simulink model "sim_tcst_2024_att_ctrl"  (R2020a)
settings: Solver=ode4  StartTime=0.0  StopTime=30.0  FixedStep=0.01  RelTol=1e-3
values from neighbouring files (symbols this model uses):
  beta0 = 2    [init_tcst_2024_att_ctrl.m]
  c1_diff_sigma_bar_w = diag([12; 12; 12])    [init_tcst_2024_att_ctrl.m]
  c1_diff_ui = diag([25; 30; 20])    [init_tcst_2024_att_ctrl.m]
  c2_diff_sigma_bar_w = diag([12; 12; 12])    [init_tcst_2024_att_ctrl.m]
  c2_diff_ui = diag([50; 50; 10])    [init_tcst_2024_att_ctrl.m]
  c3_diff_sigma_bar_w = diag([15; 15; 15])    [init_tcst_2024_att_ctrl.m]
  c3_diff_ui = diag([15; 15; 10])    [init_tcst_2024_att_ctrl.m]
  dw_aa_t = 0.2 * ones(3, 5) + ( 1.0 - 0.2 ) * rand(3, 5)    [init_tcst_2024_att_ctrl.m]
  dw_ff_t = [ 0.4 * ones(1, 5) + ( 1.0 - 0.4 ) * rand(1, 5);                      0.4 * ones(1, 5) + ( 1.0 - 0.4 ) * rand(1, 5);                      0.2 * ones(1, 5) + ( 0.6 - 0.2 ) * rand(1, 5) ]    [init_tcst_2024_att_ctrl.m]
  dw_phi_t = ( - pi / 2 ) * ones(3, 5) + ( pi / 2 - ( - pi / 2 ) ) * rand(3, 5)    [init_tcst_2024_att_ctrl.m]
  dwci_init = zeros(3,5)    [init_tcst_2024_att_ctrl.m]
  err_Ri_bar_init = zeros(3,NF)    [init_tcst_2024_att_ctrl.m]
  Fi_init = zeros(3,NF)    [init_tcst_2024_att_ctrl.m]
  h1w = diag([20.0; 20.0; 20.0])    [init_tcst_2024_att_ctrl.m]
  h2w = diag([30.0; 35.0; 35.0])    [init_tcst_2024_att_ctrl.m]
  h3w = diag([30.0; 25.0; 30.0])    [init_tcst_2024_att_ctrl.m]
  Ji = zeros(3,3,NF)    [init_tcst_2024_att_ctrl.m]
  kr1 = 10    [init_tcst_2024_att_ctrl.m]
  kr2 = 10    [init_tcst_2024_att_ctrl.m]
  kr3 = 5    [init_tcst_2024_att_ctrl.m]
  Lamd_diff_sigma_bar_w = 0.8    [init_tcst_2024_att_ctrl.m]
  Lamd_diff_ui = 0.8    [init_tcst_2024_att_ctrl.m]
  mu_d_w = 100    [init_tcst_2024_att_ctrl.m]
  pos0 = zeros(3, 1)    [init_tcst_2024_att_ctrl.m]
  PZ0 = P0(3)    [init_tcst_2024_att_ctrl.m]
  PZ1 = 10    [init_tcst_2024_att_ctrl.m]
  Qci_init = repmat([1;0;0;0],1,NF)    [init_tcst_2024_att_ctrl.m]
  Qei_init = zeros(4,NF)    [init_tcst_2024_att_ctrl.m]
  R0 = 4    [init_tcst_2024_att_ctrl.m]
  R1 = 8    [init_tcst_2024_att_ctrl.m]
  Rci_init = zeros(3,3,NF)    [init_tcst_2024_att_ctrl.m]
  Rei_init = zeros(3,3,NF)    [init_tcst_2024_att_ctrl.m]
  Ri_init = zeros(3,3,NF)    [init_tcst_2024_att_ctrl.m]
  Rx2 = 10    [init_tcst_2024_att_ctrl.m]
  Ry2 = 6    [init_tcst_2024_att_ctrl.m]
  Rz2 = 4    [init_tcst_2024_att_ctrl.m]
  T0 = 0    [init_tcst_2024_att_ctrl.m]
  T1 = tseq1    (= 10)    [init_tcst_2024_att_ctrl.m]
  T2 = tseq1 + tseq12 + tseq2    (= 30)    [init_tcst_2024_att_ctrl.m]
  ui_init = zeros(3,NF)    [init_tcst_2024_att_ctrl.m]
  V_Phi_Rei_init = zeros(3,NF)    [init_tcst_2024_att_ctrl.m]
  vel0 = zeros(3, 1)    [init_tcst_2024_att_ctrl.m]
  wci_init = zeros(3,5)    [init_tcst_2024_att_ctrl.m]
  wei_init = zeros(3,NF)    [init_tcst_2024_att_ctrl.m]
  zeta_diff_sigma_bar_w = 0.3    [init_tcst_2024_att_ctrl.m]
  zeta_diff_ui = 0.05    [init_tcst_2024_att_ctrl.m]
undefined symbols (not defined in the file or in its folder): cal_frac_squ, p_alfaw1, p_alfaw2, q_alfaw1, q_alfaw2, Qi_init, wi_init
(part 3 of 4)

== matlab function sim_tcst_2024_att_ctrl/combine wci dwci ==
  data: wci_node_1 input; wci_vec output; wci_node_2 input; wci_node_3 input; wci_node_4 input; wci_node_5 input; dwci_vec output; dwci_node_1 input; dwci_node_2 input; dwci_node_3 input; dwci_node_4 input; dwci_node_5 input
function [wci_vec, dwci_vec] = fcn(wci_node_1, wci_node_2, wci_node_3, wci_node_4, wci_node_5, ...
                                                                dwci_node_1, dwci_node_2, dwci_node_3, dwci_node_4, dwci_node_5)
%%%% 合并姿态角速率指令及其导数
wci_vec = [wci_node_1(:), wci_node_2(:), wci_node_3(:), wci_node_4(:), wci_node_5(:)];
dwci_vec = [dwci_node_1(:), dwci_node_2(:), dwci_node_3(:), dwci_node_4(:), dwci_node_5(:)];

== matlab function sim_tcst_2024_att_ctrl/cal abs 11 ==
  data: x input; y output
function y = fcn(x)
y = abs(x(:));

== matlab function sim_tcst_2024_att_ctrl/cal abs 12 ==
  data: x input; y output
function y = fcn(x)
y = abs(x(:));

== matlab function sim_tcst_2024_att_ctrl/cal abs 13 ==
  data: x input; y output
function y = fcn(x)
y = abs(x(:));

== matlab function sim_tcst_2024_att_ctrl/cal abs 14 ==
  data: x input; y output
function y = fcn(x)
y = abs(x(:));

== matlab function sim_tcst_2024_att_ctrl/cal abs 15 ==
  data: x input; y output
function y = fcn(x)
y = abs(x(:));

== matlab function sim_tcst_2024_att_ctrl/cal err_Ri_bar agent 1 ==
  data: kr1 input; err_Ri_bar_1 output; wei_vec input; V_Phi_Rei_vec input
function err_Ri_bar_1 = fcn(kr1, wei_vec, V_Phi_Rei_vec)
%%%% 计算辅助姿态旋转误差
iiuav = 1;
err_Ri_bar_1 = wei_vec(:,iiuav) + kr1 * V_Phi_Rei_vec(:,iiuav);
end

== matlab function sim_tcst_2024_att_ctrl/cal abs 16 ==
  data: x input; y output
function y = fcn(x)
y = abs(x(:));

== matlab function sim_tcst_2024_att_ctrl/cal abs 17 ==
  data: x input; y output
function y = fcn(x)
y = abs(x(:));

== matlab function sim_tcst_2024_att_ctrl/cal abs 18 ==
  data: x input; y output
function y = fcn(x)
y = abs(x(:));

== matlab function sim_tcst_2024_att_ctrl/combine tau ==
  data: tau_1 input; taui_vec output; tau_2 input; tau_3 input; tau_4 input; tau_5 input
function taui_vec = fcn(tau_1, tau_2, tau_3, tau_4, tau_5)
%%%% 合并辅助姿态角速率
taui_vec = [tau_1(:), tau_2(:), tau_3(:), tau_4(:), tau_5(:)];

== matlab function sim_tcst_2024_att_ctrl/wi dynam agent 1 ==
  data: Ji input; dwi_1 output; wi_vec input; taui_vec input; dw_vec input
function dwi_1 = fcn(Ji, wi_vec, taui_vec, dw_vec)
%%%% 更新姿态角速率微分方程
iiuav = 1;
dwi_1 = inv(Ji(:,:,iiuav)) * ( -cal_askew_mat(wi_vec(:,iiuav)) * Ji(:,:,iiuav) * wi_vec(:,iiuav) ... 
                                                + taui_vec(:,iiuav) + dw_vec(:,iiuav) );

end

== matlab function sim_tcst_2024_att_ctrl/cal abs 19 ==
  data: x input; y output
function y = fcn(x)
y = abs(x(:));

== matlab function sim_tcst_2024_att_ctrl/cal abs 20 ==
  data: x input; y output
function y = fcn(x)
y = abs(x(:));

== matlab function sim_tcst_2024_att_ctrl/cal d_sigma_w agent 1 ==
  data: h3w input; d_sigma_w_1 output; Ji input; wi_vec input; taui_vec input; sigma_w_bar_vec input
function d_sigma_w_1 = fcn(h3w, Ji, wi_vec, taui_vec, sigma_w_bar_vec)
%%%% 计算辅助姿态角速率导数
iiuav = 1;
d_sigma_w_1 = inv(Ji(:,:,iiuav)) * ( -cal_askew_mat(wi_vec(:,iiuav)) * Ji(:,:,iiuav) * wi_vec(:,iiuav) ...
                            + taui_vec(:,iiuav) + h3w * sigma_w_bar_vec(:,iiuav) );

== matlab function sim_tcst_2024_att_ctrl/cal d_sigma_w agent 2 ==
  data: h3w input; d_sigma_w_2 output; Ji input; wi_vec input; taui_vec input; sigma_w_bar_vec input
function d_sigma_w_2 = fcn(h3w, Ji, wi_vec, taui_vec, sigma_w_bar_vec)
%%%% 计算辅助姿态角速率导数
iiuav = 2;
d_sigma_w_2 = inv(Ji(:,:,iiuav)) * ( -cal_askew_mat(wi_vec(:,iiuav)) * Ji(:,:,iiuav) * wi_vec(:,iiuav) ...
                            + taui_vec(:,iiuav) + h3w * sigma_w_bar_vec(:,iiuav) );

== matlab function sim_tcst_2024_att_ctrl/cal d_sigma_w agent 3 ==
  data: h3w input; d_sigma_w_3 output; Ji input; wi_vec input; taui_vec input; sigma_w_bar_vec input
function d_sigma_w_3 = fcn(h3w, Ji, wi_vec, taui_vec, sigma_w_bar_vec)
%%%% 计算辅助姿态角速率导数
iiuav = 3;
d_sigma_w_3 = inv(Ji(:,:,iiuav)) * ( -cal_askew_mat(wi_vec(:,iiuav)) * Ji(:,:,iiuav) * wi_vec(:,iiuav) ...
                            + taui_vec(:,iiuav) + h3w * sigma_w_bar_vec(:,iiuav) );

== matlab function sim_tcst_2024_att_ctrl/cal err_Ri_bar agent 2 ==
  data: kr1 input; err_Ri_bar_2 output; wei_vec input; V_Phi_Rei_vec input
function err_Ri_bar_2 = fcn(kr1, wei_vec, V_Phi_Rei_vec)
%%%% 计算辅助姿态旋转误差
iiuav = 2;
err_Ri_bar_2 = wei_vec(:,iiuav) + kr1 * V_Phi_Rei_vec(:,iiuav);
end

== matlab function sim_tcst_2024_att_ctrl/cal d_sigma_w agent 4 ==
  data: h3w input; d_sigma_w_4 output; Ji input; wi_vec input; taui_vec input; sigma_w_bar_vec input
function d_sigma_w_4 = fcn(h3w, Ji, wi_vec, taui_vec, sigma_w_bar_vec)
%%%% 计算辅助姿态角速率导数
iiuav = 4;
d_sigma_w_4 = inv(Ji(:,:,iiuav)) * ( -cal_askew_mat(wi_vec(:,iiuav)) * Ji(:,:,iiuav) * wi_vec(:,iiuav) ...
                            + taui_vec(:,iiuav) + h3w * sigma_w_bar_vec(:,iiuav) );

== matlab function sim_tcst_2024_att_ctrl/wi dynam agent 2 ==
  data: Ji input; dwi_2 output; wi_vec input; taui_vec input; dw_vec input
function dwi_2 = fcn(Ji, wi_vec, taui_vec, dw_vec)
%%%% 更新姿态角速率微分方程
iiuav = 2;
dwi_2 = inv(Ji(:,:,iiuav)) * ( -cal_askew_mat(wi_vec(:,iiuav)) * Ji(:,:,iiuav) * wi_vec(:,iiuav) ... 
                                                + taui_vec(:,iiuav) + dw_vec(:,iiuav) );

end

== matlab function sim_tcst_2024_att_ctrl/wi dynam agent 3 ==
  data: Ji input; dwi_3 output; wi_vec input; taui_vec input; dw_vec input
function dwi_3 = fcn(Ji, wi_vec, taui_vec, dw_vec)
%%%% 更新姿态角速率微分方程
iiuav = 3;
dwi_3 = inv(Ji(:,:,iiuav)) * ( -cal_askew_mat(wi_vec(:,iiuav)) * Ji(:,:,iiuav) * wi_vec(:,iiuav) ...
                                                + taui_vec(:,iiuav) + dw_vec(:,iiuav) );

end

== matlab function sim_tcst_2024_att_ctrl/wi dynam agent 4 ==
  data: Ji input; dwi_4 output; wi_vec input; taui_vec input; dw_vec input
function dwi_4 = fcn(Ji, wi_vec, taui_vec, dw_vec)
%%%% 更新姿态角速率微分方程
iiuav = 4;
dwi_4 = inv(Ji(:,:,iiuav)) * ( -cal_askew_mat(wi_vec(:,iiuav)) * Ji(:,:,iiuav) * wi_vec(:,iiuav) ...
                                                + taui_vec(:,iiuav) + dw_vec(:,iiuav) );

end

== matlab function sim_tcst_2024_att_ctrl/wi dynam agent 5 ==
  data: Ji input; dwi_5 output; wi_vec input; taui_vec input; dw_vec input
function dwi_5 = fcn(Ji, wi_vec, taui_vec, dw_vec)
%%%% 更新姿态角速率微分方程
iiuav = 5;
dwi_5 = inv(Ji(:,:,iiuav)) * ( -cal_askew_mat(wi_vec(:,iiuav)) * Ji(:,:,iiuav) * wi_vec(:,iiuav) ...
                                                + taui_vec(:,iiuav) + dw_vec(:,iiuav) );

end

== matlab function sim_tcst_2024_att_ctrl/combine dwi ==
  data: wi_1 input; wi_vec output; wi_2 input; wi_3 input; wi_4 input; wi_5 input
function wi_vec = fcn(wi_1, wi_2, wi_3, wi_4, wi_5)
%%%% 合并姿态角速率
wi_vec = [wi_1(:), wi_2(:), wi_3(:), wi_4(:), wi_5(:)];

== matlab function sim_tcst_2024_att_ctrl/Qi dynam agent 1 ==
  data: Qi_vec input; dQi_1 output; wi_vec input
function dQi_1 = fcn(Qi_vec, wi_vec)
%%%% 更新四元数微分方程
iiuav = 1;

wi = wi_vec(:,iiuav);
thetai = Qi_vec(1,iiuav);
qi = Qi_vec(2:4,iiuav);

GammaQi = zeros(4,3);
GammaQi(1,:) = -(qi');
GammaQi(2:4,:) = thetai*eye(3,3) + cal_askew_mat(qi);
dQi_1 = (1/2)*GammaQi*wi;

end

== matlab function sim_tcst_2024_att_ctrl/Qi dynam agent 2 ==
  data: Qi_vec input; dQi_2 output; wi_vec input
function dQi_2 = fcn(Qi_vec, wi_vec)
%%%% 更新四元数微分方程
iiuav = 2;

wi = wi_vec(:,iiuav);
thetai = Qi_vec(1,iiuav);
qi = Qi_vec(2:4,iiuav);

GammaQi = zeros(4,3);
GammaQi(1,:) = -(qi');
GammaQi(2:4,:) = thetai*eye(3,3) + cal_askew_mat(qi);
dQi_2 = (1/2)*GammaQi*wi;

end

== matlab function sim_tcst_2024_att_ctrl/cal d_sigma_w agent 5 ==
  data: h3w input; d_sigma_w_5 output; Ji input; wi_vec input; taui_vec input; sigma_w_bar_vec input
function d_sigma_w_5 = fcn(h3w, Ji, wi_vec, taui_vec, sigma_w_bar_vec)
%%%% 计算辅助姿态角速率导数
iiuav = 5;
d_sigma_w_5 = inv(Ji(:,:,iiuav)) * ( -cal_askew_mat(wi_vec(:,iiuav)) * Ji(:,:,iiuav) * wi_vec(:,iiuav) ...
                            + taui_vec(:,iiuav) + h3w * sigma_w_bar_vec(:,iiuav) );

== matlab function sim_tcst_2024_att_ctrl/cal err_Ri_bar agent 3 ==
  data: kr1 input; err_Ri_bar_3 output; wei_vec input; V_Phi_Rei_vec input
function err_Ri_bar_3 = fcn(kr1, wei_vec, V_Phi_Rei_vec)
%%%% 计算辅助姿态旋转误差
iiuav = 3;
err_Ri_bar_3 = wei_vec(:,iiuav) + kr1 * V_Phi_Rei_vec(:,iiuav);
end

== matlab function sim_tcst_2024_att_ctrl/cal differentiator d_sigma_bar_w_hat agent 1/cal differentiator ==
  data: c1 input; d_sigma_bar_v_hat output; d_dsigma_bar_v_hat output; d_d2sigma_bar_v_hat output; c2 input; c3 input; chi_t input; sigma_bar_v_sig_1 input; sigma_bar_v_sig_2 input; sigma_bar_v_sig_3 input; sigma_bar_v_sig_4 input; sigma_bar_v_sig_5 input; sigma_bar_v_sig_6 input; d_sigma_bar_v_hat input; d2_sigma_bar_v_hat input
function [d_sigma_bar_v_hat, d_dsigma_bar_v_hat, d_d2sigma_bar_v_hat] = fcn(c1, c2, c3, chi_t, sigma_bar_v_sig_1, sigma_bar_v_sig_2, sigma_bar_v_sig_3, ...
                                                                                                                                                sigma_bar_v_sig_4, sigma_bar_v_sig_5, sigma_bar_v_sig_6, d_sigma_bar_v_hat, d2_sigma_bar_v_hat)
d_d2sigma_bar_v_hat = -chi_t .* c1 * sigma_bar_v_sig_1(:) - (1 - chi_t) .* c1 * sigma_bar_v_sig_2(:);
d_dsigma_bar_v_hat = -chi_t .* c2 * sigma_bar_v_sig_3(:) - (1 - chi_t) .* c2 * sigma_bar_v_sig_4(:) + d2_sigma_bar_v_hat(:);
d_sigma_bar_v_hat = -chi_t .* c3 * sigma_bar_v_sig_5(:) - (1 - chi_t) .* c3 * sigma_bar_v_sig_6(:) + d_sigma_bar_v_hat(:);

== matlab function sim_tcst_2024_att_ctrl/cal differentiator d_sigma_bar_w_hat agent 1/cal sig ==
  data: x input; z output; y input
function z = fcn(x, y)
z = x(:) .* sign(y(:));

== matlab function sim_tcst_2024_att_ctrl/cal differentiator d_sigma_bar_w_hat agent 1/cal sig1 ==
  data: x input; z output; y input
function z = fcn(x, y)
z = x(:) .* sign(y(:));

== matlab function sim_tcst_2024_att_ctrl/cal differentiator d_sigma_bar_w_hat agent 1/cal sig2 ==
  data: x input; z output; y input
function z = fcn(x, y)
z = x(:) .* sign(y(:));

== matlab function sim_tcst_2024_att_ctrl/cal differentiator d_sigma_bar_w_hat agent 1/cal sig3 ==
  data: x input; z output; y input
function z = fcn(x, y)
z = x(:) .* sign(y(:));

== matlab function sim_tcst_2024_att_ctrl/cal differentiator d_sigma_bar_w_hat agent 1/cal sig4 ==
  data: x input; z output; y input
function z = fcn(x, y)
z = x(:) .* sign(y(:));

== matlab function sim_tcst_2024_att_ctrl/cal differentiator d_sigma_bar_w_hat agent 1/cal sig5 ==
  data: x input; z output; y input
function z = fcn(x, y)
z = x(:) .* sign(y(:));

== matlab function sim_tcst_2024_att_ctrl/cal differentiator d_sigma_bar_w_hat agent 1/choose sigma_bar_w ==
  data: x input; y output
function y = fcn(x)
iiuav = 1;
y = x(:,iiuav);

== matlab function sim_tcst_2024_att_ctrl/cal differentiator d_sigma_bar_w_hat agent 1/trans to column20 ==
  data: x input; y output
function y = fcn(x)
y = x(:);

== matlab function sim_tcst_2024_att_ctrl/cal differentiator d_sigma_bar_w_hat agent 1/trans to column21 ==
  data: x input; y output
function y = fcn(x)
y = x(:);

== matlab function sim_tcst_2024_att_ctrl/cal err_Ri_bar agent 4 ==
  data: kr1 input; err_Ri_bar_4 output; wei_vec input; V_Phi_Rei_vec input
function err_Ri_bar_4 = fcn(kr1, wei_vec, V_Phi_Rei_vec)
%%%% 计算辅助姿态旋转误差
iiuav = 4;
err_Ri_bar_4 = wei_vec(:,iiuav) + kr1 * V_Phi_Rei_vec(:,iiuav);
end

== matlab function sim_tcst_2024_att_ctrl/cal differentiator d_sigma_bar_w_hat agent 1/trans to column22 ==
  data: x input; y output
function y = fcn(x)
y = x(:);

== matlab function sim_tcst_2024_att_ctrl/cal differentiator d_sigma_bar_w_hat agent 1/trans to column23 ==
  data: x input; y output
function y = fcn(x)
y = x(:);

== matlab function sim_tcst_2024_att_ctrl/cal differentiator d_sigma_bar_w_hat agent 1/trans to column24 ==
  data: x input; y output
function y = fcn(x)
y = x(:);

== matlab function sim_tcst_2024_att_ctrl/cal differentiator d_sigma_bar_w_hat agent 1/trans to column25 ==
  data: x input; y output
function y = fcn(x)
y = x(:);

== matlab function sim_tcst_2024_att_ctrl/cal differentiator d_sigma_bar_w_hat agent 2/cal differentiator ==
  data: c1 input; d_sigma_bar_v_hat output; d_dsigma_bar_v_hat output; d_d2sigma_bar_v_hat output; c2 input; c3 input; chi_t input; sigma_bar_v_sig_1 input; sigma_bar_v_sig_2 input; sigma_bar_v_sig_3 input; sigma_bar_v_sig_4 input; sigma_bar_v_sig_5 input; sigma_bar_v_sig_6 input; d_sigma_bar_v_hat input; d2_sigma_bar_v_hat input
function [d_sigma_bar_v_hat, d_dsigma_bar_v_hat, d_d2sigma_bar_v_hat] = fcn(c1, c2, c3, chi_t, sigma_bar_v_sig_1, sigma_bar_v_sig_2, sigma_bar_v_sig_3, ...
                                                                                                                                                sigma_bar_v_sig_4, sigma_bar_v_sig_5, sigma_bar_v_sig_6, d_sigma_bar_v_hat, d2_sigma_bar_v_hat)
d_d2sigma_bar_v_hat = -chi_t .* c1 * sigma_bar_v_sig_1(:) - (1 - chi_t) .* c1 * sigma_bar_v_sig_2(:);
d_dsigma_bar_v_hat = -chi_t .* c2 * sigma_bar_v_sig_3(:) - (1 - chi_t) .* c2 * sigma_bar_v_sig_4(:) + d2_sigma_bar_v_hat(:);
d_sigma_bar_v_hat = -chi_t .* c3 * sigma_bar_v_sig_5(:) - (1 - chi_t) .* c3 * sigma_bar_v_sig_6(:) + d_sigma_bar_v_hat(:);

== matlab function sim_tcst_2024_att_ctrl/cal differentiator d_sigma_bar_w_hat agent 2/cal sig ==
  data: x input; z output; y input
function z = fcn(x, y)
z = x(:) .* sign(y(:));

== matlab function sim_tcst_2024_att_ctrl/cal differentiator d_sigma_bar_w_hat agent 2/cal sig1 ==
  data: x input; z output; y input
function z = fcn(x, y)
z = x(:) .* sign(y(:));

== matlab function sim_tcst_2024_att_ctrl/cal differentiator d_sigma_bar_w_hat agent 2/cal sig2 ==
  data: x input; z output; y input
function z = fcn(x, y)
z = x(:) .* sign(y(:));

== matlab function sim_tcst_2024_att_ctrl/cal differentiator d_sigma_bar_w_hat agent 2/cal sig3 ==
  data: x input; z output; y input
function z = fcn(x, y)
z = x(:) .* sign(y(:));

== matlab function sim_tcst_2024_att_ctrl/cal differentiator d_sigma_bar_w_hat agent 2/cal sig4 ==
  data: x input; z output; y input
function z = fcn(x, y)
z = x(:) .* sign(y(:));

== matlab function sim_tcst_2024_att_ctrl/cal differentiator d_sigma_bar_w_hat agent 2/cal sig5 ==
  data: x input; z output; y input
function z = fcn(x, y)
z = x(:) .* sign(y(:));

== matlab function sim_tcst_2024_att_ctrl/depart wc5 ==
  data: y output; x input
function y = fcn(x)
y = x(:,5);

end

== matlab function sim_tcst_2024_att_ctrl/cal differentiator d_sigma_bar_w_hat agent 2/choose sigma_bar_w ==
  data: x input; y output
function y = fcn(x)
iiuav = 2;
y = x(:,iiuav);

== matlab function sim_tcst_2024_att_ctrl/cal differentiator d_sigma_bar_w_hat agent 2/trans to column20 ==
  data: x input; y output
function y = fcn(x)
y = x(:);

== matlab function sim_tcst_2024_att_ctrl/cal differentiator d_sigma_bar_w_hat agent 2/trans to column21 ==
  data: x input; y output
function y = fcn(x)
y = x(:);

== matlab function sim_tcst_2024_att_ctrl/cal differentiator d_sigma_bar_w_hat agent 2/trans to column22 ==
  data: x input; y output
function y = fcn(x)
y = x(:);

== matlab function sim_tcst_2024_att_ctrl/cal differentiator d_sigma_bar_w_hat agent 2/trans to column23 ==
  data: x input; y output
function y = fcn(x)
y = x(:);

== matlab function sim_tcst_2024_att_ctrl/cal taui agent 1 ==
  data: kr1 input; kr2 input; kr3 input; tau_1 output; Ji input; wi_vec input; wei_vec input; err_Ri_bar_vec input; Fi_vec input; VTi_vec input; dw_hat_vec input
function tau_1 = fcn(kr1, kr2, kr3, Ji, wi_vec, wei_vec, err_Ri_bar_vec, Fi_vec, VTi_vec, dw_hat_vec)
%%%% 计算用于姿态控制的驱动力矩控制输入
iiuav = 1;
tau_1 = -( kr3 + kr2 ) * err_Ri_bar_vec(:,iiuav) - kr1 * Ji(:,:,iiuav) * wei_vec(:,iiuav) ...
                + cal_askew_mat( wi_vec(:,iiuav) ) * Ji(:,:,iiuav) * wi_vec(:,iiuav) ...
                - Ji(:,:,iiuav) * Fi_vec(:,iiuav) - dw_hat_vec(:,iiuav) - VTi_vec(:,iiuav);
end

== matlab function sim_tcst_2024_att_ctrl/Qi dynam agent 3 ==
  data: Qi_vec input; dQi_3 output; wi_vec input
function dQi_3 = fcn(Qi_vec, wi_vec)
%%%% 更新四元数微分方程
iiuav = 3;

wi = wi_vec(:,iiuav);
thetai = Qi_vec(1,iiuav);
qi = Qi_vec(2:4,iiuav);

GammaQi = zeros(4,3);
GammaQi(1,:) = -(qi');
GammaQi(2:4,:) = thetai*eye(3,3) + cal_askew_mat(qi);
dQi_3 = (1/2)*GammaQi*wi;

end

== matlab function sim_tcst_2024_att_ctrl/Qi dynam agent 4 ==
  data: Qi_vec input; dQi_4 output; wi_vec input
function dQi_4 = fcn(Qi_vec, wi_vec)
%%%% 更新四元数微分方程
iiuav = 4;

wi = wi_vec(:,iiuav);
thetai = Qi_vec(1,iiuav);
qi = Qi_vec(2:4,iiuav);

GammaQi = zeros(4,3);
GammaQi(1,:) = -(qi');
GammaQi(2:4,:) = thetai*eye(3,3) + cal_askew_mat(qi);
dQi_4 = (1/2)*GammaQi*wi;

end

== matlab function sim_tcst_2024_att_ctrl/depart wc1 ==
  data: y output; x input
function y = fcn(x)
y = x(:,1);

end

== matlab function sim_tcst_2024_att_ctrl/Qi dynam agent 5 ==
  data: Qi_vec input; dQi_5 output; wi_vec input
function dQi_5 = fcn(Qi_vec, wi_vec)
%%%% 更新四元数微分方程
iiuav = 5;

wi = wi_vec(:,iiuav);
thetai = Qi_vec(1,iiuav);
qi = Qi_vec(2:4,iiuav);

GammaQi = zeros(4,3);
GammaQi(1,:) = -(qi');
GammaQi(2:4,:) = thetai*eye(3,3) + cal_askew_mat(qi);
dQi_5 = (1/2)*GammaQi*wi;

end

== matlab function sim_tcst_2024_att_ctrl/combine Qi Ri ==
  data: Qi_1 input; Qi_vec output; Qi_2 input; Qi_3 input; Qi_4 input; Qi_5 input; Ri_1 input; Ri_2 input; Ri_3 input; Ri_4 input; Ri_5 input; Ri_vec output
function [Qi_vec, Ri_vec] = fcn(Qi_1, Qi_2, Qi_3, Qi_4, Qi_5, ...
                                                        Ri_1, Ri_2, Ri_3, Ri_4, Ri_5)
%%%% 合并四元数和姿态旋转矩阵
Qi_vec = zeros(4,5);
Qi_vec(:,1) = Qi_1(:);
Qi_vec(:,2) = Qi_2(:);
Qi_vec(:,3) = Qi_3(:);
Qi_vec(:,4) = Qi_4(:);
Qi_vec(:,5) = Qi_5(:);

Ri_vec = zeros(3,3,5);
Ri_vec(:,:,1) = Ri_1;
Ri_vec(:,:,2) = Ri_2;
Ri_vec(:,:,3) = Ri_3;
Ri_vec(:,:,4) = Ri_4;
Ri_vec(:,:,5) = Ri_5;

== matlab function sim_tcst_2024_att_ctrl/cal differentiator d_sigma_bar_w_hat agent 2/trans to column24 ==
  data: x input; y output
function y = fcn(x)
y = x(:);

== matlab function sim_tcst_2024_att_ctrl/cal differentiator d_sigma_bar_w_hat agent 2/trans to column25 ==
  data: x input; y output
function y = fcn(x)
y = x(:);

== matlab function sim_tcst_2024_att_ctrl/cal differentiator d_sigma_bar_w_hat agent 3/cal differentiator ==
  data: c1 input; d_sigma_bar_v_hat output; d_dsigma_bar_v_hat output; d_d2sigma_bar_v_hat output; c2 input; c3 input; chi_t input; sigma_bar_v_sig_1 input; sigma_bar_v_sig_2 input; sigma_bar_v_sig_3 input; sigma_bar_v_sig_4 input; sigma_bar_v_sig_5 input; sigma_bar_v_sig_6 input; d_sigma_bar_v_hat input; d2_sigma_bar_v_hat input
function [d_sigma_bar_v_hat, d_dsigma_bar_v_hat, d_d2sigma_bar_v_hat] = fcn(c1, c2, c3, chi_t, sigma_bar_v_sig_1, sigma_bar_v_sig_2, sigma_bar_v_sig_3, ...
                                                                                                                                                sigma_bar_v_sig_4, sigma_bar_v_sig_5, sigma_bar_v_sig_6, d_sigma_bar_v_hat, d2_sigma_bar_v_hat)
d_d2sigma_bar_v_hat = -chi_t .* c1 * sigma_bar_v_sig_1(:) - (1 - chi_t) .* c1 * sigma_bar_v_sig_2(:);
d_dsigma_bar_v_hat = -chi_t .* c2 * sigma_bar_v_sig_3(:) - (1 - chi_t) .* c2 * sigma_bar_v_sig_4(:) + d2_sigma_bar_v_hat(:);
d_sigma_bar_v_hat = -chi_t .* c3 * sigma_bar_v_sig_5(:) - (1 - chi_t) .* c3 * sigma_bar_v_sig_6(:) + d_sigma_bar_v_hat(:);

== matlab function sim_tcst_2024_att_ctrl/cal differentiator d_sigma_bar_w_hat agent 3/cal sig ==
  data: x input; z output; y input
function z = fcn(x, y)
z = x(:) .* sign(y(:));

== matlab function sim_tcst_2024_att_ctrl/depart wc2 ==
  data: y output; x input
function y = fcn(x)
y = x(:,2);

end

== matlab function sim_tcst_2024_att_ctrl/cal differentiator d_sigma_bar_w_hat agent 3/cal sig1 ==
  data: x input; z output; y input
function z = fcn(x, y)
z = x(:) .* sign(y(:));

== matlab function sim_tcst_2024_att_ctrl/cal differentiator d_sigma_bar_w_hat agent 3/cal sig2 ==
  data: x input; z output; y input
function z = fcn(x, y)
z = x(:) .* sign(y(:));

== matlab function sim_tcst_2024_att_ctrl/cal combine sigma_bar_w_tilt ==
  data: sigma_bar_w_vec input; sigma_bar_w_hat_vec input; sigma_bar_w_tilt_vec output
function sigma_bar_w_tilt_vec = fcn(sigma_bar_w_vec, sigma_bar_w_hat_vec)
%%%% 计算虚拟速度观测误差sigma_bar_w_tilt
sigma_bar_w_tilt_vec = zeros(3,5);
for iiuav = 1:5
    sigma_bar_w_tilt_vec(:,iiuav) = sigma_bar_w_vec(:,iiuav) - sigma_bar_w_hat_vec(:,iiuav);
end

== matlab function sim_tcst_2024_att_ctrl/cal differentiator d_sigma_bar_w_hat agent 3/cal sig3 ==
  data: x input; z output; y input
function z = fcn(x, y)
z = x(:) .* sign(y(:));

== matlab function sim_tcst_2024_att_ctrl/cal differentiator d_sigma_bar_w_hat agent 3/cal sig4 ==
  data: x input; z output; y input
function z = fcn(x, y)
z = x(:) .* sign(y(:));

== matlab function sim_tcst_2024_att_ctrl/cal wei agent 1 ==
  data: wi_vec input; wei_1 output; Rei_vec input; wci_vec input
function wei_1 = fcn(wi_vec, Rei_vec, wci_vec)
%%%% 更新姿态角速率误差
iiuav = 1;
wei_1 = wi_vec(:,iiuav) - (Rei_vec(:,:,iiuav)') * wci_vec(:,iiuav);

end

== matlab function sim_tcst_2024_att_ctrl/Qei dynam agent 1 ==
  data: Qei_vec input; dQei_1 output; wei_vec input
function dQei_1 = fcn(Qei_vec, wei_vec)
%%%% 更新四元数误差微分方程
iiuav = 1;

wei = wei_vec(:,iiuav);
thetaei = Qei_vec(1,iiuav);
qei = Qei_vec(2:4,iiuav);

GammaQei = zeros(4,3);
GammaQei(1,:) = -(qei');
GammaQei(2:4,:) = thetaei*eye(3,3) + cal_askew_mat(qei);
dQei_1 = (1/2)*GammaQei*wei;

end

== matlab function sim_tcst_2024_att_ctrl/cal Rei agent 1 ==
  data: Rei_1 output; Qei_vec input
function Rei_1 = fcn(Qei_vec)
%%%% 使用罗德里格公式由四元数Qei求解Rei
iiuav = 1;
thetaei_tmp = Qei_vec(1,iiuav);
qei_tmp = Qei_vec(2:4,iiuav);
Rei_1 = ((thetaei_tmp^2) - (qei_tmp')*qei_tmp) * eye(3,3) ...
                + 2 * qei_tmp * (qei_tmp') ...
                - 2 * thetaei_tmp * cal_askew_mat(qei_tmp);

end

== matlab function sim_tcst_2024_att_ctrl/Qei dynam agent 2 ==
  data: Qei_vec input; dQei_2 output; wei_vec input
function dQei_2 = fcn(Qei_vec, wei_vec)
%%%% 更新四元数误差微分方程
iiuav = 2;

wei = wei_vec(:,iiuav);
thetaei = Qei_vec(1,iiuav);
qei = Qei_vec(2:4,iiuav);

GammaQei = zeros(4,3);
GammaQei(1,:) = -(qei');
GammaQei(2:4,:) = thetaei*eye(3,3) + cal_askew_mat(qei);
dQei_2 = (1/2)*GammaQei*wei;

end

== matlab function sim_tcst_2024_att_ctrl/depart wc3 ==
  data: y output; x input
function y = fcn(x)
y = x(:,3);

end

== matlab function sim_tcst_2024_att_ctrl/cal differentiator d_sigma_bar_w_hat agent 3/cal sig5 ==
  data: x input; z output; y input
function z = fcn(x, y)
z = x(:) .* sign(y(:));

== matlab function sim_tcst_2024_att_ctrl/cal Rei agent 2 ==
  data: Rei_2 output; Qei_vec input
function Rei_2 = fcn(Qei_vec)
%%%% 使用罗德里格公式由四元数Qei求解Rei
iiuav = 2;
thetaei_tmp = Qei_vec(1,iiuav);
qei_tmp = Qei_vec(2:4,iiuav);
Rei_2 = ((thetaei_tmp^2) - (qei_tmp')*qei_tmp) * eye(3,3) ...
                + 2 * qei_tmp * (qei_tmp') ...
                - 2 * thetaei_tmp * cal_askew_mat(qei_tmp);

end

== matlab function sim_tcst_2024_att_ctrl/cal wei agent 2 ==
  data: wi_vec input; wei_2 output; Rei_vec input; wci_vec input
function wei_2 = fcn(wi_vec, Rei_vec, wci_vec)
%%%% 更新姿态角速率误差
iiuav = 2;
wei_2 = wi_vec(:,iiuav) - (Rei_vec(:,:,iiuav)') * wci_vec(:,iiuav);

end

== matlab function sim_tcst_2024_att_ctrl/Qei dynam agent 3 ==
  data: Qei_vec input; dQei_3 output; wei_vec input
function dQei_3 = fcn(Qei_vec, wei_vec)
%%%% 更新四元数误差微分方程
iiuav = 3;

wei = wei_vec(:,iiuav);
thetaei = Qei_vec(1,iiuav);
qei = Qei_vec(2:4,iiuav);

GammaQei = zeros(4,3);
GammaQei(1,:) = -(qei');
GammaQei(2:4,:) = thetaei*eye(3,3) + cal_askew_mat(qei);
dQei_3 = (1/2)*GammaQei*wei;

end

== matlab function sim_tcst_2024_att_ctrl/cal Rei agent 3 ==
  data: Rei_3 output; Qei_vec input
function Rei_3 = fcn(Qei_vec)
%%%% 使用罗德里格公式由四元数Qei求解Rei
iiuav = 3;
thetaei_tmp = Qei_vec(1,iiuav);
qei_tmp = Qei_vec(2:4,iiuav);
Rei_3 = ((thetaei_tmp^2) - (qei_tmp')*qei_tmp) * eye(3,3) ...
                + 2 * qei_tmp * (qei_tmp') ...
                - 2 * thetaei_tmp * cal_askew_mat(qei_tmp);

end

== matlab function sim_tcst_2024_att_ctrl/cal wei agent 3 ==
  data: wi_vec input; wei_3 output; Rei_vec input; wci_vec input
function wei_3 = fcn(wi_vec, Rei_vec, wci_vec)
%%%% 更新姿态角速率误差
iiuav = 3;
wei_3 = wi_vec(:,iiuav) - (Rei_vec(:,:,iiuav)') * wci_vec(:,iiuav);

end

== matlab function sim_tcst_2024_att_ctrl/Qei dynam agent 4 ==
  data: Qei_vec input; dQei_4 output; wei_vec input
function dQei_4 = fcn(Qei_vec, wei_vec)
%%%% 更新四元数误差微分方程
iiuav = 4;

wei = wei_vec(:,iiuav);
thetaei = Qei_vec(1,iiuav);
qei = Qei_vec(2:4,iiuav);

GammaQei = zeros(4,3);
GammaQei(1,:) = -(qei');
GammaQei(2:4,:) = thetaei*eye(3,3) + cal_askew_mat(qei);
dQei_4 = (1/2)*GammaQei*wei;

end

== matlab function sim_tcst_2024_att_ctrl/cal Rei agent 4 ==
  data: Rei_4 output; Qei_vec input
function Rei_4 = fcn(Qei_vec)
%%%% 使用罗德里格公式由四元数Qei求解Rei
iiuav = 4;
thetaei_tmp = Qei_vec(1,iiuav);
qei_tmp = Qei_vec(2:4,iiuav);
Rei_4 = ((thetaei_tmp^2) - (qei_tmp')*qei_tmp) * eye(3,3) ...
                + 2 * qei_tmp * (qei_tmp') ...
                - 2 * thetaei_tmp * cal_askew_mat(qei_tmp);

end

== matlab function sim_tcst_2024_att_ctrl/cal wei agent 4 ==
  data: wi_vec input; wei_4 output; Rei_vec input; wci_vec input
function wei_4 = fcn(wi_vec, Rei_vec, wci_vec)
%%%% 更新姿态角速率误差
iiuav = 4;
wei_4 = wi_vec(:,iiuav) - (Rei_vec(:,:,iiuav)') * wci_vec(:,iiuav);

end

== matlab function sim_tcst_2024_att_ctrl/depart wc4 ==
  data: y output; x input
function y = fcn(x)
y = x(:,4);

end

== matlab function sim_tcst_2024_att_ctrl/Qei dynam agent 5 ==
  data: Qei_vec input; dQei_5 output; wei_vec input
function dQei_5 = fcn(Qei_vec, wei_vec)
%%%% 更新四元数误差微分方程
iiuav = 5;

wei = wei_vec(:,iiuav);
thetaei = Qei_vec(1,iiuav);
qei = Qei_vec(2:4,iiuav);

GammaQei = zeros(4,3);
GammaQei(1,:) = -(qei');
GammaQei(2:4,:) = thetaei*eye(3,3) + cal_askew_mat(qei);
dQei_5 = (1/2)*GammaQei*wei;

end

== matlab function sim_tcst_2024_att_ctrl/cal Rei agent 5 ==
  data: Rei_5 output; Qei_vec input
function Rei_5 = fcn(Qei_vec)
%%%% 使用罗德里格公式由四元数Qei求解Rei
iiuav = 5;
thetaei_tmp = Qei_vec(1,iiuav);
qei_tmp = Qei_vec(2:4,iiuav);
Rei_5 = ((thetaei_tmp^2) - (qei_tmp')*qei_tmp) * eye(3,3) ...
                + 2 * qei_tmp * (qei_tmp') ...
                - 2 * thetaei_tmp * cal_askew_mat(qei_tmp);

end

== matlab function sim_tcst_2024_att_ctrl/cal wei agent 5 ==
  data: wi_vec input; wei_5 output; Rei_vec input; wci_vec input
function wei_5 = fcn(wi_vec, Rei_vec, wci_vec)
%%%% 更新姿态角速率误差
iiuav = 5;
wei_5 = wi_vec(:,iiuav) - (Rei_vec(:,:,iiuav)') * wci_vec(:,iiuav);

end

== matlab function sim_tcst_2024_att_ctrl/combine wei Qei Rei ==
  data: wei_1 input; wei_vec output; wei_2 input; wei_3 input; wei_4 input; wei_5 input; Qei_1 input; Qei_2 input; Qei_3 input; Qei_4 input; Qei_5 input; Rei_1 input; Rei_2 input; Rei_3 input; Rei_4 input; Rei_5 input; Qei_vec output; Rei_vec output
function [wei_vec, Qei_vec, Rei_vec] = fcn(wei_1, wei_2, wei_3, wei_4, wei_5, ...
                                                                            Qei_1, Qei_2, Qei_3, Qei_4, Qei_5, ...
                                                                            Rei_1, Rei_2, Rei_3, Rei_4, Rei_5)
%%%% 合并姿态角速率误差/四元数误差/姿态旋转矩阵误差
wei_vec = zeros(3,5);
wei_vec(:,1) = wei_1(:);
wei_vec(:,2) = wei_2(:);
wei_vec(:,3) = wei_3(:);
wei_vec(:,4) = wei_4(:);
wei_vec(:,5) = wei_5(:);

Qei_vec = zeros(4,5);
Qei_vec(:,1) = Qei_1(:);
Qei_vec(:,2) = Qei_2(:);
Qei_vec(:,3) = Qei_3(:);
Qei_vec(:,4) = Qei_4(:);
Qei_vec(:,5) = Qei_5(:);

Rei_vec = zeros(3,3,5);
Rei_vec(:,:,1) = Rei_1;
Rei_vec(:,:,2) = Rei_2;
Rei_vec(:,:,3) = Rei_3;
Rei_vec(:,:,4) = Rei_4;
Rei_vec(:,:,5) = Rei_5;

== matlab function sim_tcst_2024_att_ctrl/cal Ri agent 1 ==
  data: Ri_1 output; Qi_vec input
function Ri_1 = fcn(Qi_vec)
%%%% 使用罗德里格公式由四元数Qi求解Ri
iiuav = 1;
thetai_tmp = Qi_vec(1,iiuav);
qi_tmp = Qi_vec(2:4,iiuav);
Ri_1 = ((thetai_tmp^2) - (qi_tmp')*qi_tmp) * eye(3,3) ...
            + 2 * qi_tmp * (qi_tmp') ...
            - 2 * thetai_tmp * cal_askew_mat(qi_tmp);

end

== matlab function sim_tcst_2024_att_ctrl/cal Ri agent 2 ==
  data: Ri_2 output; Qi_vec input
function Ri_2 = fcn(Qi_vec)
%%%% 使用罗德里格公式由四元数Qi求解Ri
iiuav = 2;
thetai_tmp = Qi_vec(1,iiuav);
qi_tmp = Qi_vec(2:4,iiuav);
Ri_2 = ((thetai_tmp^2) - (qi_tmp')*qi_tmp) * eye(3,3) ...
            + 2 * qi_tmp * (qi_tmp') ...
            - 2 * thetai_tmp * cal_askew_mat(qi_tmp);

end

== matlab function sim_tcst_2024_att_ctrl/cal Ri agent 3 ==
  data: Ri_3 output; Qi_vec input
function Ri_3 = fcn(Qi_vec)
%%%% 使用罗德里格公式由四元数Qi求解Ri
iiuav = 3;
thetai_tmp = Qi_vec(1,iiuav);
qi_tmp = Qi_vec(2:4,iiuav);
Ri_3 = ((thetai_tmp^2) - (qi_tmp')*qi_tmp) * eye(3,3) ...
            + 2 * qi_tmp * (qi_tmp') ...
            - 2 * thetai_tmp * cal_askew_mat(qi_tmp);

end

== matlab function sim_tcst_2024_att_ctrl/depart Qc5 ==
  data: y output; x input
function y = fcn(x)
y = x(:,5);

end

== matlab function sim_tcst_2024_att_ctrl/cal Ri agent 4 ==
  data: Ri_4 output; Qi_vec input
function Ri_4 = fcn(Qi_vec)
%%%% 使用罗德里格公式由四元数Qi求解Ri
iiuav = 4;
thetai_tmp = Qi_vec(1,iiuav);
qi_tmp = Qi_vec(2:4,iiuav);
Ri_4 = ((thetai_tmp^2) - (qi_tmp')*qi_tmp) * eye(3,3) ...
            + 2 * qi_tmp * (qi_tmp') ...
            - 2 * thetai_tmp * cal_askew_mat(qi_tmp);

end

== matlab function sim_tcst_2024_att_ctrl/cal Ri agent 5 ==
  data: Ri_5 output; Qi_vec input
function Ri_5 = fcn(Qi_vec)
%%%% 使用罗德里格公式由四元数Qi求解Ri
iiuav = 5;
thetai_tmp = Qi_vec(1,iiuav);
qi_tmp = Qi_vec(2:4,iiuav);
Ri_5 = ((thetai_tmp^2) - (qi_tmp')*qi_tmp) * eye(3,3) ...
            + 2 * qi_tmp * (qi_tmp') ...
            - 2 * thetai_tmp * cal_askew_mat(qi_tmp);

end

== matlab function sim_tcst_2024_att_ctrl/cal Qci agent 1 ==
  data: Qi_vec input; Qci_1 output; Qei_vec input
function Qci_1 = fcn(Qi_vec, Qei_vec)
%%%% 更新期望指令四元数
iiuav = 1;

sigma1 = Qi_vec(1,iiuav);
q1 = Qi_vec(2:4,iiuav);
sigma2 = Qei_vec(1,iiuav);
q2 = -Qei_vec(2:4,iiuav);

sigma = sigma1*sigma2 - (q1')*q2;
q = sigma1*q2 + sigma2*q1 + cal_askew_mat(q1)*q2;
Qci_1 = [sigma; q];

end

== matlab function sim_tcst_2024_att_ctrl/cal Rci agent 1 ==
  data: Rci_1 output; Qci input
function Rci_1 = fcn(Qci)
%%%% 使用罗德里格公式由四元数Qci求解Rci
thetaci_tmp = Qci(1,1);
qci_tmp = Qci(2:4,1);
Rci_1 = ((thetaci_tmp^2) - (qci_tmp')*qci_tmp) * eye(3,3) ...
                + 2 * qci_tmp * (qci_tmp') ...
                - 2 * thetaci_tmp * cal_askew_mat(qci_tmp);

end

== matlab function sim_tcst_2024_att_ctrl/cal Qci agent 2 ==
  data: Qi_vec input; Qci_2 output; Qei_vec input
function Qci_2 = fcn(Qi_vec, Qei_vec)
%%%% 更新期望指令四元数
iiuav = 2;
sigma1 = Qi_vec(1,iiuav);
q1 = Qi_vec(2:4,iiuav);
sigma2 = Qei_vec(1,iiuav);
q2 = -Qei_vec(2:4,iiuav);

sigma = sigma1*sigma2 - (q1')*q2;
q = sigma1*q2 + sigma2*q1 + cal_askew_mat(q1)*q2;
Qci_2 = [sigma; q];

end

== matlab function sim_tcst_2024_att_ctrl/cal Rci agent 2 ==
  data: Rci_2 output; Qci input
function Rci_2 = fcn(Qci)
%%%% 使用罗德里格公式由四元数Qci求解Rci

thetaci_tmp = Qci(1,1);
qci_tmp = Qci(2:4,1);
Rci_2 = ((thetaci_tmp^2) - (qci_tmp')*qci_tmp) * eye(3,3) ...
                + 2 * qci_tmp * (qci_tmp') ...
                - 2 * thetaci_tmp * cal_askew_mat(qci_tmp);

end

== matlab function sim_tcst_2024_att_ctrl/cal Qci agent 3 ==
  data: Qi_vec input; Qci_3 output; Qei_vec input
function Qci_3 = fcn(Qi_vec, Qei_vec)
%%%% 更新期望指令四元数
iiuav = 3;
sigma1 = Qi_vec(1,iiuav);
q1 = Qi_vec(2:4,iiuav);
sigma2 = Qei_vec(1,iiuav);
q2 = -Qei_vec(2:4,iiuav);

sigma = sigma1*sigma2 - (q1')*q2;
q = sigma1*q2 + sigma2*q1 + cal_askew_mat(q1)*q2;
Qci_3 = [sigma; q];

end

== matlab function sim_tcst_2024_att_ctrl/cal Rci agent 3 ==
  data: Rci_3 output; Qci input
function Rci_3 = fcn(Qci)
%%%% 使用罗德里格公式由四元数Qci求解Rci
thetaci_tmp = Qci(1,1);
qci_tmp = Qci(2:4,1);
Rci_3 = ((thetaci_tmp^2) - (qci_tmp')*qci_tmp) * eye(3,3) ...
                + 2 * qci_tmp * (qci_tmp') ...
                - 2 * thetaci_tmp * cal_askew_mat(qci_tmp);

end

== matlab function sim_tcst_2024_att_ctrl/cal Qci agent 4 ==
  data: Qi_vec input; Qci_4 output; Qei_vec input
function Qci_4 = fcn(Qi_vec, Qei_vec)
%%%% 更新期望指令四元数
iiuav = 4;
sigma1 = Qi_vec(1,iiuav);
q1 = Qi_vec(2:4,iiuav);
sigma2 = Qei_vec(1,iiuav);
q2 = -Qei_vec(2:4,iiuav);

sigma = sigma1*sigma2 - (q1')*q2;
q = sigma1*q2 + sigma2*q1 + cal_askew_mat(q1)*q2;
Qci_4 = [sigma; q];

end

== matlab function sim_tcst_2024_att_ctrl/cal Rci agent 4 ==
  data: Rci_4 output; Qci input
function Rci_4 = fcn(Qci)
%%%% 使用罗德里格公式由四元数Qci求解Rci
thetaci_tmp = Qci(1,1);
qci_tmp = Qci(2:4,1);
Rci_4 = ((thetaci_tmp^2) - (qci_tmp')*qci_tmp) * eye(3,3) ...
                + 2 * qci_tmp * (qci_tmp') ...
                - 2 * thetaci_tmp * cal_askew_mat(qci_tmp);

end

== matlab function sim_tcst_2024_att_ctrl/depart Qc1 ==
  data: y output; x input
function y = fcn(x)
y = x(:,1);

end

== matlab function sim_tcst_2024_att_ctrl/cal Qci agent 5 ==
  data: Qi_vec input; Qci_5 output; Qei_vec input
function Qci_5 = fcn(Qi_vec, Qei_vec)
%%%% 更新期望指令四元数
iiuav = 5;
sigma1 = Qi_vec(1,iiuav);
q1 = Qi_vec(2:4,iiuav);
sigma2 = Qei_vec(1,iiuav);
q2 = -Qei_vec(2:4,iiuav);

sigma = sigma1*sigma2 - (q1')*q2;
q = sigma1*q2 + sigma2*q1 + cal_askew_mat(q1)*q2;
Qci_5 = [sigma; q];

end

== matlab function sim_tcst_2024_att_ctrl/cal Rci agent 5 ==
  data: Rci_5 output; Qci_vec input
function Rci_5 = fcn(Qci_vec)
%%%% 使用罗德里格公式由四元数Qci求解Rci
thetaci_tmp = Qci_vec(1,1);
qci_tmp = Qci_vec(2:4,1);
Rci_5 = ((thetaci_tmp^2) - (qci_tmp')*qci_tmp) * eye(3,3) ...
                + 2 * qci_tmp * (qci_tmp') ...
                - 2 * thetaci_tmp * cal_askew_mat(qci_tmp);

end

== matlab function sim_tcst_2024_att_ctrl/combine Qci Rci ==
  data: Qci_1 input; Qci_vec output; Qci_2 input; Qci_3 input; Qci_4 input; Qci_5 input; Rci_1 input; Rci_2 input; Rci_3 input; Rci_4 input; Rci_5 input; Rci_vec output
function [Qci_vec, Rci_vec] = fcn(Qci_1, Qci_2, Qci_3, Qci_4, Qci_5, ...
                                                            Rci_1, Rci_2, Rci_3, Rci_4, Rci_5)
%%%% 合并四元数和姿态旋转矩阵
Qci_vec = zeros(4,5);
Qci_vec(:,1) = Qci_1(:);
Qci_vec(:,2) = Qci_2(:);
Qci_vec(:,3) = Qci_3(:);
Qci_vec(:,4) = Qci_4(:);
Qci_vec(:,5) = Qci_5(:);

Rci_vec = zeros(3,3,5);
Rci_vec(:,:,1) = Rci_1;
Rci_vec(:,:,2) = Rci_2;
Rci_vec(:,:,3) = Rci_3;
Rci_vec(:,:,4) = Rci_4;
Rci_vec(:,:,5) = Rci_5;

== matlab function sim_tcst_2024_att_ctrl/cal differentiator d_sigma_bar_w_hat agent 3/choose sigma_bar_w ==
  data: x input; y output
function y = fcn(x)
iiuav = 3;
y = x(:,iiuav);

== matlab function sim_tcst_2024_att_ctrl/cal differentiator d_sigma_bar_w_hat agent 3/trans to column20 ==
  data: x input; y output
function y = fcn(x)
y = x(:);

== matlab function sim_tcst_2024_att_ctrl/cal differentiator d_sigma_bar_w_hat agent 3/trans to column21 ==
  data: x input; y output
function y = fcn(x)
y = x(:);

== matlab function sim_tcst_2024_att_ctrl/cal differentiator d_sigma_bar_w_hat agent 3/trans to column22 ==
  data: x input; y output
function y = fcn(x)
y = x(:);

== matlab function sim_tcst_2024_att_ctrl/cal differentiator d_sigma_bar_w_hat agent 3/trans to column23 ==
  data: x input; y output
function y = fcn(x)
y = x(:);

== matlab function sim_tcst_2024_att_ctrl/depart Qc2 ==
  data: y output; x input
function y = fcn(x)
y = x(:,2);

end

== matlab function sim_tcst_2024_att_ctrl/combine Qci Rci1 ==
  data: V_Phi_Rei_1 input; V_Phi_Rei_vec output; V_Phi_Rei_2 input; V_Phi_Rei_3 input; V_Phi_Rei_4 input; V_Phi_Rei_5 input
function V_Phi_Rei_vec = fcn(V_Phi_Rei_1, V_Phi_Rei_2, V_Phi_Rei_3, V_Phi_Rei_4, V_Phi_Rei_5)
%%%% 合并LogSO3空间的辅助姿态误差向量
V_Phi_Rei_vec = [V_Phi_Rei_1(:), V_Phi_Rei_2(:), V_Phi_Rei_3(:), V_Phi_Rei_4(:), V_Phi_Rei_5(:)];

== matlab function sim_tcst_2024_att_ctrl/depart Qe1 ==
  data: y output; x input
function y = fcn(x)
y = x(:,1);

end

== matlab function sim_tcst_2024_att_ctrl/depart Qe2 ==
  data: y output; x input
function y = fcn(x)
y = x(:,2);

end

== matlab function sim_tcst_2024_att_ctrl/depart Qe3 ==
  data: y output; x input
function y = fcn(x)
y = x(:,3);

end

== matlab function sim_tcst_2024_att_ctrl/depart Qe4 ==
  data: y output; x input
function y = fcn(x)
y = x(:,4);

end

== matlab function sim_tcst_2024_att_ctrl/depart Qe5 ==
  data: y output; x input
function y = fcn(x)
y = x(:,5);

end

== matlab function sim_tcst_2024_att_ctrl/depart we1 ==
  data: y output; x input
function y = fcn(x)
y = x(:,1);

end

== matlab function sim_tcst_2024_att_ctrl/depart we2 ==
  data: y output; x input
function y = fcn(x)
y = x(:,2);

end

== matlab function sim_tcst_2024_att_ctrl/depart we3 ==
  data: y output; x input
function y = fcn(x)
y = x(:,3);

end

== matlab function sim_tcst_2024_att_ctrl/depart Qc3 ==
  data: y output; x input
function y = fcn(x)
y = x(:,3);

end

== matlab function sim_tcst_2024_att_ctrl/depart we4 ==
  data: y output; x input
function y = fcn(x)
y = x(:,4);

end

== matlab function sim_tcst_2024_att_ctrl/depart we5 ==
  data: y output; x input
function y = fcn(x)
y = x(:,5);

end

== matlab function sim_tcst_2024_att_ctrl/depart V_Phi_Re5 ==
  data: y output; x input
function y = fcn(x)
y = x(:,5);

end

== matlab function sim_tcst_2024_att_ctrl/depart V_Phi_Re1 ==
  data: y output; x input
function y = fcn(x)
y = x(:,1);

end

== matlab function sim_tcst_2024_att_ctrl/depart V_Phi_Re2 ==
  data: y output; x input
function y = fcn(x)
y = x(:,2);

end

== matlab function sim_tcst_2024_att_ctrl/depart V_Phi_Re3 ==
  data: y output; x input
function y = fcn(x)
y = x(:,3);

end

== matlab function sim_tcst_2024_att_ctrl/depart V_Phi_Re4 ==
  data: y output; x input
function y = fcn(x)
y = x(:,4);

end

== matlab function sim_tcst_2024_att_ctrl/cal differentiator d_sigma_bar_w_hat agent 3/trans to column24 ==
  data: x input; y output
function y = fcn(x)
y = x(:);

== matlab function sim_tcst_2024_att_ctrl/cal differentiator d_sigma_bar_w_hat agent 3/trans to column25 ==
  data: x input; y output
function y = fcn(x)
y = x(:);

== matlab function sim_tcst_2024_att_ctrl/cal differentiator d_sigma_bar_w_hat agent 4/cal differentiator ==
  data: c1 input; d_sigma_bar_v_hat output; d_dsigma_bar_v_hat output; d_d2sigma_bar_v_hat output; c2 input; c3 input; chi_t input; sigma_bar_v_sig_1 input; sigma_bar_v_sig_2 input; sigma_bar_v_sig_3 input; sigma_bar_v_sig_4 input; sigma_bar_v_sig_5 input; sigma_bar_v_sig_6 input; d_sigma_bar_v_hat input; d2_sigma_bar_v_hat input
function [d_sigma_bar_v_hat, d_dsigma_bar_v_hat, d_d2sigma_bar_v_hat] = fcn(c1, c2, c3, chi_t, sigma_bar_v_sig_1, sigma_bar_v_sig_2, sigma_bar_v_sig_3, ...
                                                                                                                                                sigma_bar_v_sig_4, sigma_bar_v_sig_5, sigma_bar_v_sig_6, d_sigma_bar_v_hat, d2_sigma_bar_v_hat)
d_d2sigma_bar_v_hat = -chi_t .* c1 * sigma_bar_v_sig_1(:) - (1 - chi_t) .* c1 * sigma_bar_v_sig_2(:);
d_dsigma_bar_v_hat = -chi_t .* c2 * sigma_bar_v_sig_3(:) - (1 - chi_t) .* c2 * sigma_bar_v_sig_4(:) + d2_sigma_bar_v_hat(:);
d_sigma_bar_v_hat = -chi_t .* c3 * sigma_bar_v_sig_5(:) - (1 - chi_t) .* c3 * sigma_bar_v_sig_6(:) + d_sigma_bar_v_hat(:);

== matlab function sim_tcst_2024_att_ctrl/depart Qc4 ==
  data: y output; x input
function y = fcn(x)
y = x(:,4);

end

== matlab function sim_tcst_2024_att_ctrl/cal differentiator d_sigma_bar_w_hat agent 4/cal sig ==
  data: x input; z output; y input
function z = fcn(x, y)
z = x(:) .* sign(y(:));

== matlab function sim_tcst_2024_att_ctrl/cal differentiator d_sigma_bar_w_hat agent 4/cal sig1 ==
  data: x input; z output; y input
function z = fcn(x, y)
z = x(:) .* sign(y(:));

== matlab function sim_tcst_2024_att_ctrl/cal differentiator d_sigma_bar_w_hat agent 4/cal sig2 ==
  data: x input; z output; y input
function z = fcn(x, y)
z = x(:) .* sign(y(:));

== matlab function sim_tcst_2024_att_ctrl/cal differentiator d_sigma_bar_w_hat agent 4/cal sig3 ==
  data: x input; z output; y input
function z = fcn(x, y)
z = x(:) .* sign(y(:));

== matlab function sim_tcst_2024_att_ctrl/cal differentiator d_sigma_bar_w_hat agent 4/cal sig4 ==
  data: x input; z output; y input
function z = fcn(x, y)
z = x(:) .* sign(y(:));

== matlab function sim_tcst_2024_att_ctrl/cal differentiator d_sigma_bar_w_hat agent 4/cal sig5 ==
  data: x input; z output; y input
function z = fcn(x, y)
z = x(:) .* sign(y(:));

== matlab function sim_tcst_2024_att_ctrl/cal differentiator d_sigma_bar_w_hat agent 4/choose sigma_bar_w ==
  data: x input; y output
function y = fcn(x)
iiuav = 4;
y = x(:,iiuav);

== matlab function sim_tcst_2024_att_ctrl/cal differentiator d_sigma_bar_w_hat agent 4/trans to column20 ==
  data: x input; y output
function y = fcn(x)
y = x(:);

== matlab function sim_tcst_2024_att_ctrl/cal err_Ri_bar agent 5 ==
  data: kr1 input; err_Ri_bar_5 output; wei_vec input; V_Phi_Rei_vec input
function err_Ri_bar_5 = fcn(kr1, wei_vec, V_Phi_Rei_vec)
%%%% 计算辅助姿态旋转误差
iiuav = 5;
err_Ri_bar_5 = wei_vec(:,iiuav) + kr1 * V_Phi_Rei_vec(:,iiuav);
end

== matlab function sim_tcst_2024_att_ctrl/cal differentiator d_sigma_bar_w_hat agent 4/trans to column21 ==
  data: x input; y output
function y = fcn(x)
y = x(:);

== matlab function sim_tcst_2024_att_ctrl/cal differentiator d_sigma_bar_w_hat agent 4/trans to column22 ==
  data: x input; y output
function y = fcn(x)
y = x(:);

== matlab function sim_tcst_2024_att_ctrl/cal differentiator d_sigma_bar_w_hat agent 4/trans to column23 ==
  data: x input; y output
function y = fcn(x)
y = x(:);

== matlab function sim_tcst_2024_att_ctrl/cal differentiator d_sigma_bar_w_hat agent 4/trans to column24 ==
  data: x input; y output
function y = fcn(x)
y = x(:);

== matlab function sim_tcst_2024_att_ctrl/cal differentiator d_sigma_bar_w_hat agent 4/trans to column25 ==
  data: x input; y output
function y = fcn(x)
y = x(:);

== matlab function sim_tcst_2024_att_ctrl/cal differentiator d_sigma_bar_w_hat agent 5/cal differentiator ==
  data: c1 input; d_sigma_bar_v_hat output; d_dsigma_bar_v_hat output; d_d2sigma_bar_v_hat output; c2 input; c3 input; chi_t input; sigma_bar_v_sig_1 input; sigma_bar_v_sig_2 input; sigma_bar_v_sig_3 input; sigma_bar_v_sig_4 input; sigma_bar_v_sig_5 input; sigma_bar_v_sig_6 input; d_sigma_bar_v_hat input; d2_sigma_bar_v_hat input
function [d_sigma_bar_v_hat, d_dsigma_bar_v_hat, d_d2sigma_bar_v_hat] = fcn(c1, c2, c3, chi_t, sigma_bar_v_sig_1, sigma_bar_v_sig_2, sigma_bar_v_sig_3, ...
                                                                                                                                                sigma_bar_v_sig_4, sigma_bar_v_sig_5, sigma_bar_v_sig_6, d_sigma_bar_v_hat, d2_sigma_bar_v_hat)
d_d2sigma_bar_v_hat = -chi_t .* c1 * sigma_bar_v_sig_1(:) - (1 - chi_t) .* c1 * sigma_bar_v_sig_2(:);
d_dsigma_bar_v_hat = -chi_t .* c2 * sigma_bar_v_sig_3(:) - (1 - chi_t) .* c2 * sigma_bar_v_sig_4(:) + d2_sigma_bar_v_hat(:);
d_sigma_bar_v_hat = -chi_t .* c3 * sigma_bar_v_sig_5(:) - (1 - chi_t) .* c3 * sigma_bar_v_sig_6(:) + d_sigma_bar_v_hat(:);

== matlab function sim_tcst_2024_att_ctrl/cal differentiator d_sigma_bar_w_hat agent 5/cal sig ==
  data: x input; z output; y input
function z = fcn(x, y)
z = x(:) .* sign(y(:));

== matlab function sim_tcst_2024_att_ctrl/cal differentiator d_sigma_bar_w_hat agent 5/cal sig1 ==
  data: x input; z output; y input
function z = fcn(x, y)
z = x(:) .* sign(y(:));

== matlab function sim_tcst_2024_att_ctrl/cal differentiator d_sigma_bar_w_hat agent 5/cal sig2 ==
  data: x input; z output; y input
function z = fcn(x, y)
z = x(:) .* sign(y(:));

== matlab function sim_tcst_2024_att_ctrl/cal differentiator d_sigma_bar_w_hat agent 5/cal sig3 ==
  data: x input; z output; y input
function z = fcn(x, y)
z = x(:) .* sign(y(:));

== matlab function sim_tcst_2024_att_ctrl/combine err_Ri_bar ==
  data: err_Ri_bar_1 input; err_Ri_bar_vec output; err_Ri_bar_2 input; err_Ri_bar_3 input; err_Ri_bar_4 input; err_Ri_bar_5 input
function err_Ri_bar_vec = fcn(err_Ri_bar_1, err_Ri_bar_2, err_Ri_bar_3, err_Ri_bar_4, err_Ri_bar_5)
%%%% 合并辅助姿态旋转误差向量
err_Ri_bar_vec = [err_Ri_bar_1(:), err_Ri_bar_2(:), err_Ri_bar_3(:), err_Ri_bar_4(:), err_Ri_bar_5(:)];

== matlab function sim_tcst_2024_att_ctrl/cal differentiator d_sigma_bar_w_hat agent 5/cal sig4 ==
  data: x input; z output; y input
function z = fcn(x, y)
z = x(:) .* sign(y(:));

== matlab function sim_tcst_2024_att_ctrl/cal differentiator d_sigma_bar_w_hat agent 5/cal sig5 ==
  data: x input; z output; y input
function z = fcn(x, y)
z = x(:) .* sign(y(:));

== matlab function sim_tcst_2024_att_ctrl/cal differentiator d_sigma_bar_w_hat agent 5/choose sigma_bar_w ==
  data: x input; y output
function y = fcn(x)
iiuav = 5;
y = x(:,iiuav);

== matlab function sim_tcst_2024_att_ctrl/cal differentiator d_sigma_bar_w_hat agent 5/trans to column20 ==
  data: x input; y output
function y = fcn(x)
y = x(:);

== matlab function sim_tcst_2024_att_ctrl/cal differentiator d_sigma_bar_w_hat agent 5/trans to column21 ==
  data: x input; y output
function y = fcn(x)
y = x(:);

== matlab function sim_tcst_2024_att_ctrl/cal differentiator d_sigma_bar_w_hat agent 5/trans to column22 ==
  data: x input; y output
function y = fcn(x)
y = x(:);

== matlab function sim_tcst_2024_att_ctrl/cal differentiator d_sigma_bar_w_hat agent 5/trans to column23 ==
  data: x input; y output
function y = fcn(x)
y = x(:);

== matlab function sim_tcst_2024_att_ctrl/cal differentiator d_sigma_bar_w_hat agent 5/trans to column24 ==
  data: x input; y output
function y = fcn(x)
y = x(:);

== matlab function sim_tcst_2024_att_ctrl/cal differentiator d_sigma_bar_w_hat agent 5/trans to column25 ==
  data: x input; y output
function y = fcn(x)
y = x(:);

== matlab function sim_tcst_2024_att_ctrl/cal dw_hat agent 1 ==
  data: h3w input; Ji input; d_sigma_bar_w_vec input; sigma_bar_w_hat_vec input; dw_hat_1 output
function dw_hat_1 = fcn(h3w, Ji, d_sigma_bar_w_vec, sigma_bar_w_hat_vec)
%%%% 计算扰动观测值dw_hat
iiuav = 1;
dw_hat_1 = Ji(:,:,iiuav) * d_sigma_bar_w_vec(:,iiuav) + h3w * sigma_bar_w_hat_vec(:,iiuav);

== matlab function sim_tcst_2024_att_ctrl/cal dw_hat agent 2 ==
  data: h3w input; Ji input; d_sigma_bar_w_vec input; sigma_bar_w_hat_vec input; dw_hat_2 output
function dw_hat_2 = fcn(h3w, Ji, d_sigma_bar_w_vec, sigma_bar_w_hat_vec)
%%%% 计算扰动观测值dw_hat
iiuav = 2;
dw_hat_2 = Ji(:,:,iiuav) * d_sigma_bar_w_vec(:,iiuav) + h3w * sigma_bar_w_hat_vec(:,iiuav);
